simulink model "Propulsor"  (R2024a)
settings: Solver=FixedStepAuto  StartTime=0.0  StopTime=tf  FixedStep=step_modelo  RelTol=1e-3
values from neighbouring files (symbols this model uses):
  Fn = inp.Fn(i)    [RCS_Entradas.m]
  mib = inp.mib(i)    [RCS_Entradas.m]
  tc = inp.tc(i)    [RCS_Entradas.m]
  Td = inp.Td(i)    [RCS_Entradas.m]
  Tpulse = inp.Tpulse(i)    [RCS_Entradas.m]
undefined symbols (not defined in the file or in its folder): peak_prop
libraries: simulink x1, dspsrcs4 x1
settings Model: PacingRate=0.100000  Creator=rodri  LastModifiedBy=rodri
settings DataIOCC: SaveOutput=off  SaveTime=off
settings RTWCC: GPUComputeCapability=3.5

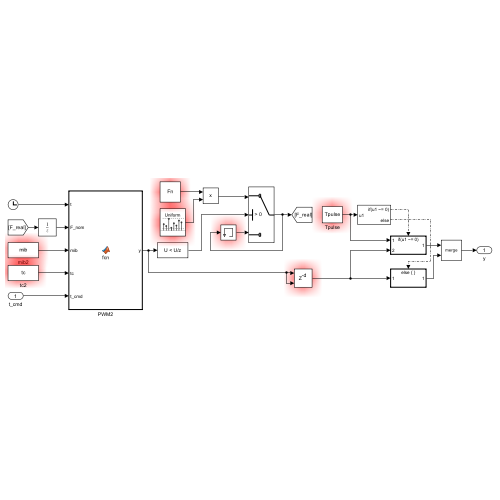
[thumbnail: Simulink's stored preview of the top-level diagram]
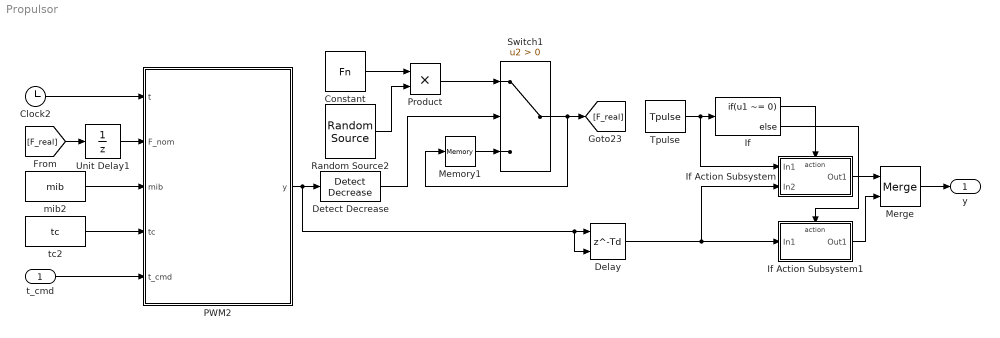
== system Propulsor ==
  t_cmd : Inport  OutDataTypeStr=double  PortDimensions=1
  Clock2 : Clock
  Constant : Constant  Value=Fn  SampleTime=-1
  Delay : Delay  DelayLength=Td  InitialConditionSource=Input port  InitialCondition=0
      settings: InputPortMap=u0,p4
  Detect Decrease : simulink/Logic and Bit Operations/Detect Decrease  vinit=0.0  OutDataTypeStr=boolean
  If : If  IfExpression=u1 ~= 0
  If Action Subsystem : Subsystem  TreatAsAtomicUnit=on
  If Action Subsystem1 : Subsystem  TreatAsAtomicUnit=on
  Memory1 : Memory  InitialCondition=Fn  InheritSampleTime=on
  Merge : Merge
  PWM2 : MATLAB Function  TreatAsAtomicUnit=on
  Product : Product
  Random Source2 : dspsrcs4/Random Source  SrcType=Uniform  MinVal=1-peak_prop/100  MaxVal=1+peak_prop/100  MeanVal=0  VarVal=1  RepMode=Not repeatable  rawSeed=1  IsInherit=off  SampTime=step_modelo  SampFrame=1  OutComplex=Real  DataType=double  SimulateUsing=Code generation
  Switch1 : Switch  Criteria=u2 > Threshold  SaturateOnIntegerOverflow=off  InputSameDT=off
  Tpulse : Constant  Value=Tpulse  SampleTime=-1
  Unit Delay1 : UnitDelay  SampleTime=-1  HasFrameUpgradeWarning=on
  mib2 : Constant  Value=mib  SampleTime=-1
  tc2 : Constant  Value=tc  SampleTime=-1
  y : Outport  OutDataTypeStr=double  PortDimensions=1
  wires:
  Clock2/1 -> PWM2/1(t)
  t_cmd/1 -> PWM2/5(t_cmd)
  tc2/1 -> PWM2/4(tc)
  mib2/1 -> PWM2/3(mib)
  Unit Delay1/1 -> PWM2/2(F_nom)
  Constant/1 -> Product/1
  Detect Decrease/1 -> Switch1/2
  Switch1/1 -> Memory1/1, [F_real]
  Random Source2/1 -> Product/2
  Product/1 -> Switch1/1
  Memory1/1 -> Switch1/3
  [F_real] -> Unit Delay1/1
  Tpulse/1 -> If Action Subsystem/1(In1), If/1
  PWM2/1(y) -> Delay/2, Delay/1, Detect Decrease/1
  If Action Subsystem1/1(Out1) -> Merge/2
  If/1 -> If Action Subsystem/Action
  If/2 -> If Action Subsystem1/Action
  Delay/1 -> If Action Subsystem1/1(In1), If Action Subsystem/2(In2)
  Merge/1 -> y/1
  If Action Subsystem/1(Out1) -> Merge/1

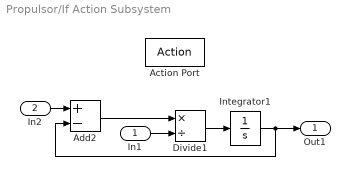
== system Propulsor/If Action Subsystem ==
  In1 : Inport
  In2 : Inport  Port=2
  Action Port : ActionPort  ActionPortLabel=if(u1 ~= 0)
  Add2 : Sum  Inputs=+-
  Divide1 : Product  Inputs=*/
  Integrator1 : Integrator
  Out1 : Outport
  wires:
  In2/1 -> Add2/1
  Integrator1/1 -> Out1/1, Add2/2
  Add2/1 -> Divide1/1
  Divide1/1 -> Integrator1/1
  In1/1 -> Divide1/2

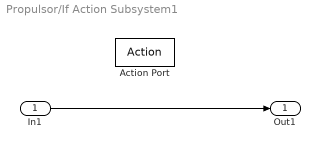
== system Propulsor/If Action Subsystem1 ==
  In1 : Inport
  Action Port : ActionPort  ActionPortLabel=else
  Out1 : Outport
  wires:
  In1/1 -> Out1/1

== matlab function Propulsor/PWM2 ==
  data: t input; F_nom input; mib input; tc input; y output; t_cmd input
function y  = fcn(t,F_nom,mib,tc,t_cmd)

%Ciclo de controle.
control_cycle = 1/tc;

%Tempo mínimo de acionamento do propulsor dado o seu mib.
tmin = mib/F_nom;

if tmin >= t_cmd %Lógica para desprezar entradas de tempo menores que o mib. 
    y = 0;
else
    %Fdes é a força desejada pelo sistema, sendo a multiplicação do tempo de
    %acionamento (calculado e input da função) e a força nominal do propulsor.
    Fdes = t_cmd*F_nom;

    %t_acio é o tempo de acionamento do propulsor, considerando um um propulsor
    %fornece sua força nominal (F_nom) em um dado período de tempo (tc).
    t_acio = Fdes*tc/F_nom;

    %duty é a representação da porcentagem de atuação do atuador dado o período
    %de tempo tc;
    duty = t_acio*100/tc;

    %Cálculo da força fornecida em um dado período de tempo tc.
    y = F_nom*square(2*pi*control_cycle.*t,duty);
    if y <= 0
        y = 0;
    end
end
